simulink model "KW2_Q4_P2"  (R2018b)
settings: Solver=VariableStepAuto  StartTime=0.0  StopTime=100.0  RelTol=1e-3
settings Model: Creator=mohammadreza  LastModifiedBy=mohammadreza

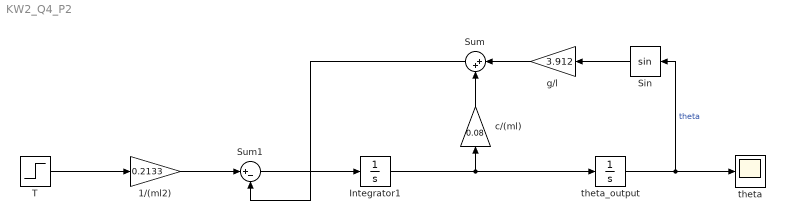
== system KW2_Q4_P2 ==
  1/(ml2) : Gain  Gain=0.2133
  Integrator1 : Integrator
  Sin : Trigonometry
  Sum : Sum  Inputs=|++
  Sum1 : Sum  Inputs=|+-
  T : Step  After=200  SampleTime=0
  c/(ml) : Gain  Gain=0.08
  g/l : Gain  Gain=3.912
  theta : Scope
  theta_output : Integrator
  wires:
  T/1 -> 1/(ml2)/1
  1/(ml2)/1 -> Sum1/1
  Sum1/1 -> Integrator1/1
  Integrator1/1 -> c/(ml)/1, theta_output/1
  c/(ml)/1 -> Sum/2
  g/l/1 -> Sum/1
  Sum/1 -> Sum1/2
  Sin/1 -> g/l/1
  theta_output/1 -> theta/1, Sin/1  "theta"
